simulink model "piezo_sim"  (R2021b)
settings: Solver=FixedStepAuto  StartTime=0.0  StopTime=4  FixedStep=tsamp  MaxStep=1e-3
values from neighbouring files (symbols this model uses):
  c = 0.2    [piezo_example.m]    (also in piezo_plant.m = x(2); piezo_reference.m = x(2); time_array.mat = 0.8)
  piezo_gain = 1e-7    (= 1e-07)    [piezo_example.m]    (also in piezo_plant.m = x(4); piezo_reference.m = x(4); time_array.mat)
  tsamp = 0.1    [gain_test.m]    (also in piezo_example.m = 0.001)
settings Model: Creator=mvanmeer  LastModifiedBy=20191777
settings SolverCC: AlgebraicLoopSolver=TrustRegion
settings DebuggingCC: UnconnectedInputMsg=none  UnconnectedOutputMsg=none  UnconnectedLineMsg=none  ArithmeticOperatorsInVariantConditions=warning
settings ModelReferenceCC: EnableRefExpFcnMdlSchedulingChecks=off
settings SFSimCC: CustomCodeUndefinedFunction=UseInterfaceOnly

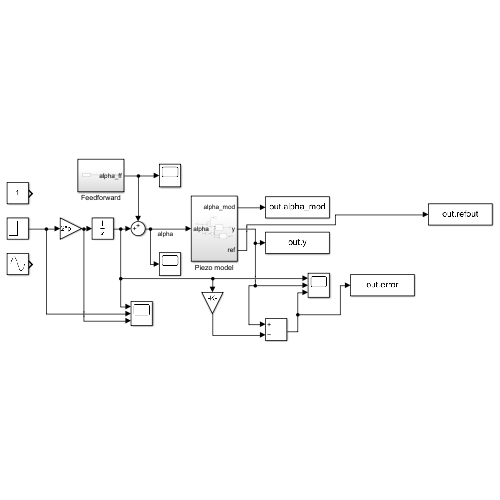
[thumbnail: Simulink's stored preview of the top-level diagram]
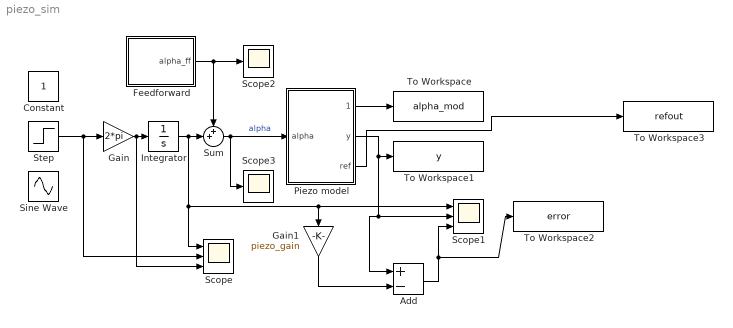
== system piezo_sim ==
  Add : Sum  Inputs=+-
  Constant : Constant
  Feedforward : Subsystem
  Gain : Gain  Gain=2*pi
  Gain1 : Gain  Gain=piezo_gain
  Integrator : Integrator
  Piezo model : Subsystem
  Scope : Scope  NumInputPorts=3
  Scope1 : Scope  NumInputPorts=3
  Scope2 : Scope
  Scope3 : Scope
  Sine Wave : Sin  Bias=0.75  Frequency=2*pi  Phase=-0.5*pi  SampleTime=0
  Step : Step  Time=2  Before=1  After=2  SampleTime=0
  Sum : Sum  Inputs=++|
  To Workspace : ToWorkspace  VariableName=alpha_mod  SaveFormat=Timeseries  SampleTime=-1
  To Workspace1 : ToWorkspace  VariableName=y  SaveFormat=Timeseries  SampleTime=-1
  To Workspace2 : ToWorkspace  VariableName=error  SaveFormat=Timeseries  SampleTime=-1
  To Workspace3 : ToWorkspace  VariableName=refout  SaveFormat=Timeseries  SampleTime=-1
  wires:
  Step/1 -> Scope/2, Gain/1
  Feedforward/1(alpha_ff) -> Sum/1, Scope2/1
  Sum/1 -> Scope3/1, Piezo model/1(alpha)  "alpha"
  Piezo model/1(alpha_mod) -> To Workspace/1
  Piezo model/2(y) -> Scope1/2, Add/1, To Workspace1/1
  Integrator/1 -> Gain1/1, Scope1/1, Scope/1, Sum/2
  Gain/1 -> Scope/3, Integrator/1
  Add/1 -> To Workspace2/1, Scope1/3
  Gain1/1 -> Add/2
  Piezo model/3(ref) -> To Workspace3/1

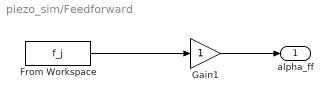
== system piezo_sim/Feedforward ==
  From Workspace : FromWorkspace  VariableName=f_j  SampleTime=tsamp
  Gain1 : Gain
  alpha_ff : Outport
  wires:
  From Workspace/1 -> Gain1/1
  Gain1/1 -> alpha_ff/1

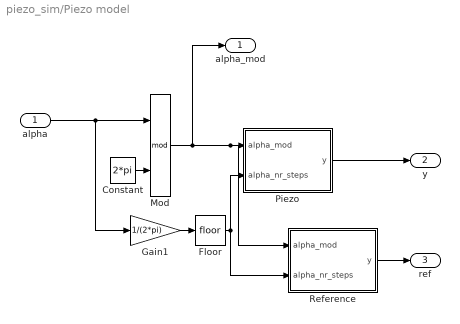
== system piezo_sim/Piezo model ==
  alpha : Inport
  Constant : Constant  Value=2*pi
  Floor : Rounding
  Gain1 : Gain  Gain=1/(2*pi)
  Mod : Math  Operator=mod  SignedPower=on  SaturateOnIntegerOverflow=on
  "Piezo " : Subsystem
  Reference : Subsystem
  alpha_mod : Outport
  y : Outport  Port=2
  ref : Outport  Port=3
  wires:
  alpha/1 -> Gain1/1, Mod/1
  Constant/1 -> Mod/2
  Floor/1 -> Reference/2(alpha_nr_steps), "Piezo "/2(alpha_nr_steps)
  Mod/1 -> alpha_mod/1, Reference/1(alpha_mod), "Piezo "/1(alpha_mod)
  Gain1/1 -> Floor/1
  "Piezo "/1(y) -> y/1
  Reference/1(y) -> ref/1

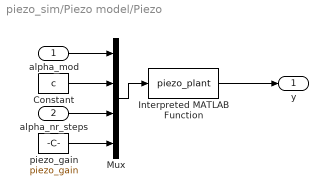
== system piezo_sim/Piezo model/Piezo  ==
  alpha_mod : Inport
  alpha_nr_steps : Inport  Port=2
  Constant : Constant  Value=c
  Interpreted MATLAB Function : MATLABFcn  MATLABFcn=piezo_plant
  Mux : Mux
  piezo_gain : Constant  Value=piezo_gain
  y : Outport
  wires:
  alpha_mod/1 -> Mux/1
  Interpreted MATLAB Function/1 -> y/1
  Mux/1 -> Interpreted MATLAB Function/1
  Constant/1 -> Mux/2
  alpha_nr_steps/1 -> Mux/3
  piezo_gain/1 -> Mux/4

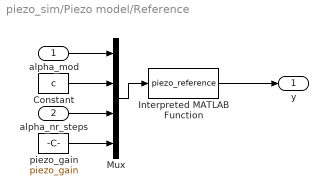
== system piezo_sim/Piezo model/Reference ==
  alpha_mod : Inport
  alpha_nr_steps : Inport  Port=2
  Constant : Constant  Value=c
  Interpreted MATLAB Function : MATLABFcn  MATLABFcn=piezo_reference
  Mux : Mux
  piezo_gain : Constant  Value=piezo_gain
  y : Outport
  wires:
  alpha_mod/1 -> Mux/1
  Interpreted MATLAB Function/1 -> y/1
  Mux/1 -> Interpreted MATLAB Function/1
  Constant/1 -> Mux/2
  alpha_nr_steps/1 -> Mux/3
  piezo_gain/1 -> Mux/4
